simulink model "MultiGain"  (R2019b)
settings: Solver=VariableStepAuto  StartTime=0.0  StopTime=10.0  RelTol=1e-3
undefined symbols (not defined in the file or in its folder): Klqr1, Klqr2, Klqr3, Klqr4, Klqr5
settings Model: Creator=alelu  LastModifiedBy=FedeB

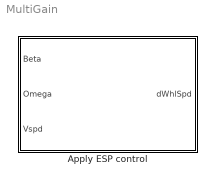
== system MultiGain ==
  Apply ESP control : Subsystem

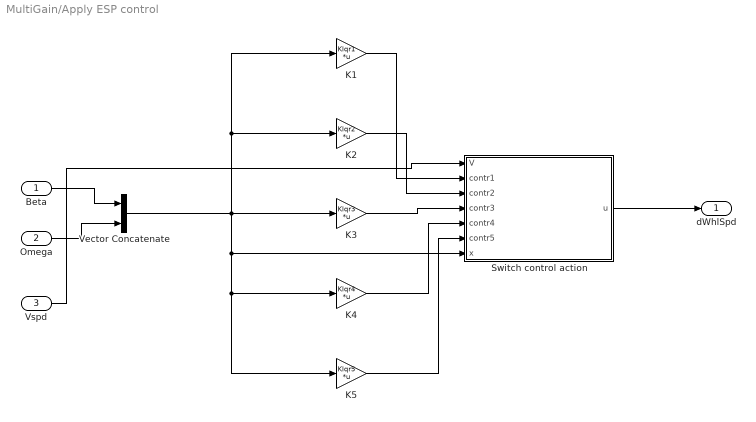
== system MultiGain/Apply ESP control ==
  Beta : Inport
  Omega : Inport  Port=2
  Vspd : Inport  Port=3
  K1 : Gain  Gain=Klqr1  Multiplication=Matrix(K*u)
  K2 : Gain  Gain=Klqr2  Multiplication=Matrix(K*u)
  K3 : Gain  Gain=Klqr3  Multiplication=Matrix(K*u)
  K4 : Gain  Gain=Klqr4  Multiplication=Matrix(K*u)
  K5 : Gain  Gain=Klqr5  Multiplication=Matrix(K*u)
  Switch control action : MATLAB Function  TreatAsAtomicUnit=on
  Vector Concatenate : Concatenate
  dWhlSpd : Outport
  wires:
  Beta/1 -> Vector Concatenate/1
  Vector Concatenate/1 -> K4/1, K5/1, Switch control action/7(x), K3/1, K2/1, K1/1
  K5/1 -> Switch control action/6(contr5)
  Omega/1 -> Vector Concatenate/2
  K1/1 -> Switch control action/2(contr1)
  K3/1 -> Switch control action/4(contr3)
  K4/1 -> Switch control action/5(contr4)
  K2/1 -> Switch control action/3(contr2)
  Vspd/1 -> Switch control action/1(V)
  Switch control action/1(u) -> dWhlSpd/1

== matlab function MultiGain/Apply ESP control/Switch control action ==
  data: V input; contr1 input; u output; contr2 input; contr3 input; contr4 input; contr5 input; x input
function u = switch_control(V, contr1, contr2, contr3, contr4, contr5, x)

%Velocities that will define our 5 possible scenarios
V1 = 60/3.6;
V2 = 80/3.6;
V3 = 100/3.6;
V4 = 120/3.6;

beta = x(1);
beta1 = beta - floor((beta+pi)/(2*pi))*(2*pi); %unwrapping of beta: brings beta back in range [-pi;pi]
w = x(2);

%Initialization of control action u
u = [0; 0; 0; 0];

if (abs(beta1) > pi/2) || (abs(w) > 4*pi)
    %if beta and omega are out of range, then do nothing
else
    switch V
        case V <= V1
            u = contr1;
        case (V > V1) && (V <= V2)
            u = contr2;
        case (V > V2) && (V <= V3)
            u = contr3;
        case (V > V3) && (V <= V4)
            u = contr4;
        case V > V4
            u = contr5;
    end
    %otherwise, select the best control action for the vehicle based on its
    %current velocity V
end
